simulink model "Example"  (R2025a)
settings: Solver=VariableStepAuto  StartTime=0.0  StopTime=100  RelTol=1e-3
PostLoadFcn:
  | TP_prop = Generate_TP_Prop('E:\refprop10\REFPROP','R134a',0.001,5.5,80,510,100,25,25);
  | TL_prop = Generate_TL_Prop('E:\refprop10\REFPROP','Water',0.01,50,273.16,373.16,20,20);
undefined symbols (not defined in the file): nu_liq, nu_vap, p, s_liq, s_vap, u_sat_liq, u_sat_vap
libraries: fl_lib x62, nesl_utility x34, SimscapeFluids_lib x28
(part 3 of 3)

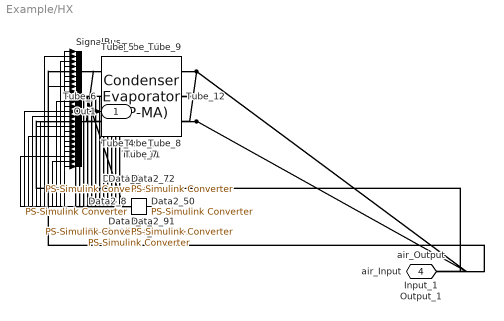
== system Example/HX ==
  Data1_{1..12} (12 alike) : nesl_utility/PS-Simulink Converter  PhysicalDomain=network_engine_domain  SubClassName=ps_output  LeftPortType=input  RightPortType=output  PseudoPeriodic=off  Frequencies=[]  VectorFormat=inherit  Unit=inherit  AffineConversion=off
  Data2_{1..12} (12 alike) : nesl_utility/PS-Simulink Converter  PhysicalDomain=network_engine_domain  SubClassName=ps_output  LeftPortType=input  RightPortType=output  PseudoPeriodic=off  Frequencies=[]  VectorFormat=inherit  Unit=inherit  AffineConversion=off
  SignalBus : BusCreator  Inputs=24
  Tube_1 : SimscapeFluids_lib/Heat Exchangers/Two-Phase Fluid - Moist Air/Condenser Evaporator (2P-MA)  flow_arrangement=fluids.heat_exchangers.enum.FlowArrangement2PMA.Cross  cross_flow_arrangement=fluids.heat_exchangers.enum.CrossFlowArrangement2PMA.UnmixedUnmixed  R_wall=1000*log(Tube_outer_diameter/Tube_inner_diameter)/(2*pi*Length_tube_segment*380) K/kW  wall_thermal_mass=false  mass_wall=1 kg  cp_wall=490 J/(K*kg)  area_A1=Cross_sectional_area_A1 m^2  area_B1=pi*Tube_inner_diameter^2/4 m^2  area_A2=Cross_sectional_area_A2/4 m^2  area_B2=Cross_sectional_area_B2/4 m^2  tube_num_2P=1  tube_length_2P=Total_length_each_tube m  tube_cross_section_2P=fluids.heat_exchangers.enum.TubeCrossSection.Circular  tube_diameter_2P=Tube_inner_diameter m  tube_width_2P=0.05 m  tube_height_2P=0.05 m  tube_inner_diameter_2P=0.05 m  tube_outer_diameter_2P=0.1 m  tube_flow_area_2P=0.002 m^2  tube_wetted_perimeter_2P=0.15 m  tube_heat_perimeter_2P=0.15 m  tube_pressure_loss_spec_2P=fluids.heat_exchangers.enum.TubePressureLossSpec2P.Haaland  tube_loss_coeff_2P=10  tube_local_pressure_loss_spec_2P=fluids.heat_exchangers.enum.LocalLossSpec.AggregateLength  tube_length_add_2P=Agg_equiv_length m  tube_local_loss_coefficient_2P=0.1  tube_roughness_pressure_2P=Internal_surface_roughness m  tube_Re_lam_pressure_2P=2000  tube_Re_tur_pressure_2P=4000  tube_shape_factor_generic_2P=64  tube_heat_coeff_spec_2P=fluids.heat_exchangers.enum.TubeHeatCoeffSpec2P.GneilinskiCavalliniZecchin  tube_colburn_coeff_liq_2P=[.023, .8, .33]  tube_colburn_coeff_mix_2P=[.05, .8, .33]  tube_colburn_coeff_vap_2P=[.023, .8, .33]  tube_roughness_heat_2P=15e-6 m  tube_Re_lam_heat_2P=2000  tube_Re_tur_heat_2P=4000  tube_Nu_lam_generic_2P=3.66  fouling_factor_2P=0.1 K*m^2/kW  fin_area_2P=0 m^2  fin_efficiency_2P=0.5  energy_spec_2P=foundation.enum.energy_spec.temperature  p_init_2P=Initial_pressure MPa  T_init_2P=Initial_temperature K  x_init_2P=0.5  alpha_init_2P=0.5  h_init_2P=1500 kJ/kg  u_init_2P=1500 kJ/kg  flow_geometry_MA=fluids.heat_exchangers.enum.FlowGeometryMA.AcrossTubeBank  tube_num_MA=25  tube_length_MA=1 m  tube_cross_section_MA=fluids.heat_exchangers.enum.TubeCrossSection.Circular  tube_diameter_MA=0.05 m  tube_width_MA=0.05 m  tube_height_MA=0.05 m  tube_inner_diameter_MA=0.05 m  tube_outer_diameter_MA=0.1 m  tube_flow_area_MA=0.002 m^2  tube_wetted_perimeter_MA=0.15 m  tube_heat_perimeter_MA=0.15 m  tube_pressure_loss_spec_MA=fluids.heat_exchangers.enum.TubePressureLossSpec.Haaland  tube_loss_coeff_MA=10  tube_local_pressure_loss_spec_MA=fluids.heat_exchangers.enum.LocalLossSpec.AggregateLength  tube_length_add_MA=0.1 m  tube_local_loss_coefficient_MA=0.1  tube_roughness_pressure_MA=15e-6 m  tube_Re_lam_pressure_MA=2000  tube_Re_tur_pressure_MA=4000  tube_shape_factor_generic_MA=64  tube_heat_coeff_spec_MA=fluids.heat_exchangers.enum.TubeHeatCoeffSpec.Gneilinski  tube_colburn_coeff_MA=[.023, .8, .33]  tube_roughness_heat_MA=15e-6 m  tube_Re_lam_heat_MA=2000  tube_Re_tur_heat_MA=4000  tube_Nu_lam_generic_MA=3.66  bank_arrangement_MA=fluids.heat_exchangers.enum.BankArrangement.Inline  bank_num_rows_MA=1  bank_tubes_per_row_MA=1  bank_width_MA=Length_tube_segment m  bank_tube_diameter_MA=Tube_outer_diameter m  bank_longitudinal_pitch_MA=Longitudinal_tube_pitch m  bank_transverse_pitch_MA=Transverse_tube_pitch m  bank_pressure_loss_spec_MA=fluids.heat_exchangers.enum.BankPressureLossSpec.Martin  bank_euler_MA=10  bank_heat_coeff_spec_MA=fluids.heat_exchangers.enum.BankHeatCoeffSpec.Martin  bank_colburn_coeff_MA=[.27, .63, .36]  generic_flow_area_MA=0.01 m^2  generic_heat_area_MA=2 m^2  generic_volume_MA=0.05 m^3  generic_loss_coeff_MA=10  generic_colburn_coeff_MA=[.023, .8, .33]  fouling_factor_MA=Fouling_factor_air K*m^2/kW  fin_area_MA=Total_fin_surface_area_air m^2  fin_efficiency_MA=Fin_efficiency_air  p_init_MA=Initial_pressure_air MPa  T_init_MA=Initial_temperature_air K  humidity_spec_MA=foundation.enum.HumiditySpec.RelativeHumidity  RH_init_MA=Initial_rel_humidity  x_w_init_MA=0.01  y_w_init_MA=0.01  HR_init_MA=0.01  Tw_init_MA=287 K  trace_gas_spec_MA=foundation.enum.trace_gas_spec.mass_fraction  x_g_init_MA=0.001  y_g_init_MA=0.001  r_d_init_MA=0  RH_ws_MA=1  time_constant_cond_MA=1e-3 s  time_constant_evap_MA=1e-3 s  fraction_entrained_MA=1
      settings: InternalSimscapePortConfiguration="{\"Bottom\":[],\"Left\":[{\"id\":\"A1\",\"label\":\"A1\",\"type\":\"foundation.two_phase_fluid.two_phase_fluid\"},{\"id\":\"Z\",\"label\":\"Z\",\"type\":\"output\"},{\"id\":\"B1\",\"label\":\"B1\",\"type\":\"foundation.two_phase_fluid.two_phase_fluid\"}],\"Right\":[{\"id\":\"A2\",\"label\":\"A2\",\"type\":\"foundation.moist_air.moist_air\"},{\"id\":\"W\",\"label\":\"W\",\"type\":\"output\"},{\"id\":\"B2\",\"label\":\"B2\",\"type\":\"foundation.moist_air.moist_air\"}],\"Top\":[]}"
  Tube_{2..11} (10 alike) : SimscapeFluids_lib/Heat Exchangers/Two-Phase Fluid - Moist Air/Condenser Evaporator (2P-MA)  flow_arrangement=fluids.heat_exchangers.enum.FlowArrangement2PMA.Cross  cross_flow_arrangement=fluids.heat_exchangers.enum.CrossFlowArrangement2PMA.UnmixedUnmixed  R_wall=1000*log(Tube_outer_diameter/Tube_inner_diameter)/(2*pi*Length_tube_segment*380) K/kW  wall_thermal_mass=false  mass_wall=1 kg  cp_wall=490 J/(K*kg)  area_A1=pi*Tube_inner_diameter^2/4 m^2  area_B1=pi*Tube_inner_diameter^2/4 m^2  area_A2=Cross_sectional_area_A2/4 m^2  area_B2=Cross_sectional_area_B2/4 m^2  tube_num_2P=1  tube_length_2P=Total_length_each_tube m  tube_cross_section_2P=fluids.heat_exchangers.enum.TubeCrossSection.Circular  tube_diameter_2P=Tube_inner_diameter m  tube_width_2P=0.05 m  tube_height_2P=0.05 m  tube_inner_diameter_2P=0.05 m  tube_outer_diameter_2P=0.1 m  tube_flow_area_2P=0.002 m^2  tube_wetted_perimeter_2P=0.15 m  tube_heat_perimeter_2P=0.15 m  tube_pressure_loss_spec_2P=fluids.heat_exchangers.enum.TubePressureLossSpec2P.Haaland  tube_loss_coeff_2P=10  tube_local_pressure_loss_spec_2P=fluids.heat_exchangers.enum.LocalLossSpec.AggregateLength  tube_length_add_2P=Agg_equiv_length m  tube_local_loss_coefficient_2P=0.1  tube_roughness_pressure_2P=Internal_surface_roughness m  tube_Re_lam_pressure_2P=2000  tube_Re_tur_pressure_2P=4000  tube_shape_factor_generic_2P=64  tube_heat_coeff_spec_2P=fluids.heat_exchangers.enum.TubeHeatCoeffSpec2P.GneilinskiCavalliniZecchin  tube_colburn_coeff_liq_2P=[.023, .8, .33]  tube_colburn_coeff_mix_2P=[.05, .8, .33]  tube_colburn_coeff_vap_2P=[.023, .8, .33]  tube_roughness_heat_2P=15e-6 m  tube_Re_lam_heat_2P=2000  tube_Re_tur_heat_2P=4000  tube_Nu_lam_generic_2P=3.66  fouling_factor_2P=0.1 K*m^2/kW  fin_area_2P=0 m^2  fin_efficiency_2P=0.5  energy_spec_2P=foundation.enum.energy_spec.temperature  p_init_2P=Initial_pressure MPa  T_init_2P=Initial_temperature K  x_init_2P=0.5  alpha_init_2P=0.5  h_init_2P=1500 kJ/kg  u_init_2P=1500 kJ/kg  flow_geometry_MA=fluids.heat_exchangers.enum.FlowGeometryMA.AcrossTubeBank  tube_num_MA=25  tube_length_MA=1 m  tube_cross_section_MA=fluids.heat_exchangers.enum.TubeCrossSection.Circular  tube_diameter_MA=0.05 m  tube_width_MA=0.05 m  tube_height_MA=0.05 m  tube_inner_diameter_MA=0.05 m  tube_outer_diameter_MA=0.1 m  tube_flow_area_MA=0.002 m^2  tube_wetted_perimeter_MA=0.15 m  tube_heat_perimeter_MA=0.15 m  tube_pressure_loss_spec_MA=fluids.heat_exchangers.enum.TubePressureLossSpec.Haaland  tube_loss_coeff_MA=10  tube_local_pressure_loss_spec_MA=fluids.heat_exchangers.enum.LocalLossSpec.AggregateLength  tube_length_add_MA=0.1 m  tube_local_loss_coefficient_MA=0.1  tube_roughness_pressure_MA=15e-6 m  tube_Re_lam_pressure_MA=2000  tube_Re_tur_pressure_MA=4000  tube_shape_factor_generic_MA=64  tube_heat_coeff_spec_MA=fluids.heat_exchangers.enum.TubeHeatCoeffSpec.Gneilinski  tube_colburn_coeff_MA=[.023, .8, .33]  tube_roughness_heat_MA=15e-6 m  tube_Re_lam_heat_MA=2000  tube_Re_tur_heat_MA=4000  tube_Nu_lam_generic_MA=3.66  bank_arrangement_MA=fluids.heat_exchangers.enum.BankArrangement.Inline  bank_num_rows_MA=1  bank_tubes_per_row_MA=1  bank_width_MA=Length_tube_segment m  bank_tube_diameter_MA=Tube_outer_diameter m  bank_longitudinal_pitch_MA=Longitudinal_tube_pitch m  bank_transverse_pitch_MA=Transverse_tube_pitch m  bank_pressure_loss_spec_MA=fluids.heat_exchangers.enum.BankPressureLossSpec.Martin  bank_euler_MA=10  bank_heat_coeff_spec_MA=fluids.heat_exchangers.enum.BankHeatCoeffSpec.Martin  bank_colburn_coeff_MA=[.27, .63, .36]  generic_flow_area_MA=0.01 m^2  generic_heat_area_MA=2 m^2  generic_volume_MA=0.05 m^3  generic_loss_coeff_MA=10  generic_colburn_coeff_MA=[.023, .8, .33]  fouling_factor_MA=Fouling_factor_air K*m^2/kW  fin_area_MA=Total_fin_surface_area_air m^2  fin_efficiency_MA=Fin_efficiency_air  p_init_MA=Initial_pressure_air MPa  T_init_MA=Initial_temperature_air K  humidity_spec_MA=foundation.enum.HumiditySpec.RelativeHumidity  RH_init_MA=Initial_rel_humidity  x_w_init_MA=0.01  y_w_init_MA=0.01  HR_init_MA=0.01  Tw_init_MA=287 K  trace_gas_spec_MA=foundation.enum.trace_gas_spec.mass_fraction  x_g_init_MA=0.001  y_g_init_MA=0.001  r_d_init_MA=0  RH_ws_MA=1  time_constant_cond_MA=1e-3 s  time_constant_evap_MA=1e-3 s  fraction_entrained_MA=1
      settings: InternalSimscapePortConfiguration="{\"Bottom\":[],\"Left\":[{\"id\":\"A1\",\"label\":\"A1\",\"type\":\"foundation.two_phase_fluid.two_phase_fluid\"},{\"id\":\"Z\",\"label\":\"Z\",\"type\":\"output\"},{\"id\":\"B1\",\"label\":\"B1\",\"type\":\"foundation.two_phase_fluid.two_phase_fluid\"}],\"Right\":[{\"id\":\"A2\",\"label\":\"A2\",\"type\":\"foundation.moist_air.moist_air\"},{\"id\":\"W\",\"label\":\"W\",\"type\":\"output\"},{\"id\":\"B2\",\"label\":\"B2\",\"type\":\"foundation.moist_air.moist_air\"}],\"Top\":[]}"
  Tube_12 : SimscapeFluids_lib/Heat Exchangers/Two-Phase Fluid - Moist Air/Condenser Evaporator (2P-MA)  flow_arrangement=fluids.heat_exchangers.enum.FlowArrangement2PMA.Cross  cross_flow_arrangement=fluids.heat_exchangers.enum.CrossFlowArrangement2PMA.UnmixedUnmixed  R_wall=1000*log(Tube_outer_diameter/Tube_inner_diameter)/(2*pi*Length_tube_segment*380) K/kW  wall_thermal_mass=false  mass_wall=1 kg  cp_wall=490 J/(K*kg)  area_A1=pi*Tube_inner_diameter^2/4 m^2  area_B1=Cross_sectional_area_B1 m^2  area_A2=Cross_sectional_area_A2/4 m^2  area_B2=Cross_sectional_area_B2/4 m^2  tube_num_2P=1  tube_length_2P=Total_length_each_tube m  tube_cross_section_2P=fluids.heat_exchangers.enum.TubeCrossSection.Circular  tube_diameter_2P=Tube_inner_diameter m  tube_width_2P=0.05 m  tube_height_2P=0.05 m  tube_inner_diameter_2P=0.05 m  tube_outer_diameter_2P=0.1 m  tube_flow_area_2P=0.002 m^2  tube_wetted_perimeter_2P=0.15 m  tube_heat_perimeter_2P=0.15 m  tube_pressure_loss_spec_2P=fluids.heat_exchangers.enum.TubePressureLossSpec2P.Haaland  tube_loss_coeff_2P=10  tube_local_pressure_loss_spec_2P=fluids.heat_exchangers.enum.LocalLossSpec.AggregateLength  tube_length_add_2P=Agg_equiv_length m  tube_local_loss_coefficient_2P=0.1  tube_roughness_pressure_2P=Internal_surface_roughness m  tube_Re_lam_pressure_2P=2000  tube_Re_tur_pressure_2P=4000  tube_shape_factor_generic_2P=64  tube_heat_coeff_spec_2P=fluids.heat_exchangers.enum.TubeHeatCoeffSpec2P.GneilinskiCavalliniZecchin  tube_colburn_coeff_liq_2P=[.023, .8, .33]  tube_colburn_coeff_mix_2P=[.05, .8, .33]  tube_colburn_coeff_vap_2P=[.023, .8, .33]  tube_roughness_heat_2P=15e-6 m  tube_Re_lam_heat_2P=2000  tube_Re_tur_heat_2P=4000  tube_Nu_lam_generic_2P=3.66  fouling_factor_2P=0.1 K*m^2/kW  fin_area_2P=0 m^2  fin_efficiency_2P=0.5  energy_spec_2P=foundation.enum.energy_spec.temperature  p_init_2P=Initial_pressure MPa  T_init_2P=Initial_temperature K  x_init_2P=0.5  alpha_init_2P=0.5  h_init_2P=1500 kJ/kg  u_init_2P=1500 kJ/kg  flow_geometry_MA=fluids.heat_exchangers.enum.FlowGeometryMA.AcrossTubeBank  tube_num_MA=25  tube_length_MA=1 m  tube_cross_section_MA=fluids.heat_exchangers.enum.TubeCrossSection.Circular  tube_diameter_MA=0.05 m  tube_width_MA=0.05 m  tube_height_MA=0.05 m  tube_inner_diameter_MA=0.05 m  tube_outer_diameter_MA=0.1 m  tube_flow_area_MA=0.002 m^2  tube_wetted_perimeter_MA=0.15 m  tube_heat_perimeter_MA=0.15 m  tube_pressure_loss_spec_MA=fluids.heat_exchangers.enum.TubePressureLossSpec.Haaland  tube_loss_coeff_MA=10  tube_local_pressure_loss_spec_MA=fluids.heat_exchangers.enum.LocalLossSpec.AggregateLength  tube_length_add_MA=0.1 m  tube_local_loss_coefficient_MA=0.1  tube_roughness_pressure_MA=15e-6 m  tube_Re_lam_pressure_MA=2000  tube_Re_tur_pressure_MA=4000  tube_shape_factor_generic_MA=64  tube_heat_coeff_spec_MA=fluids.heat_exchangers.enum.TubeHeatCoeffSpec.Gneilinski  tube_colburn_coeff_MA=[.023, .8, .33]  tube_roughness_heat_MA=15e-6 m  tube_Re_lam_heat_MA=2000  tube_Re_tur_heat_MA=4000  tube_Nu_lam_generic_MA=3.66  bank_arrangement_MA=fluids.heat_exchangers.enum.BankArrangement.Inline  bank_num_rows_MA=1  bank_tubes_per_row_MA=1  bank_width_MA=Length_tube_segment m  bank_tube_diameter_MA=Tube_outer_diameter m  bank_longitudinal_pitch_MA=Longitudinal_tube_pitch m  bank_transverse_pitch_MA=Transverse_tube_pitch m  bank_pressure_loss_spec_MA=fluids.heat_exchangers.enum.BankPressureLossSpec.Martin  bank_euler_MA=10  bank_heat_coeff_spec_MA=fluids.heat_exchangers.enum.BankHeatCoeffSpec.Martin  bank_colburn_coeff_MA=[.27, .63, .36]  generic_flow_area_MA=0.01 m^2  generic_heat_area_MA=2 m^2  generic_volume_MA=0.05 m^3  generic_loss_coeff_MA=10  generic_colburn_coeff_MA=[.023, .8, .33]  fouling_factor_MA=Fouling_factor_air K*m^2/kW  fin_area_MA=Total_fin_surface_area_air m^2  fin_efficiency_MA=Fin_efficiency_air  p_init_MA=Initial_pressure_air MPa  T_init_MA=Initial_temperature_air K  humidity_spec_MA=foundation.enum.HumiditySpec.RelativeHumidity  RH_init_MA=Initial_rel_humidity  x_w_init_MA=0.01  y_w_init_MA=0.01  HR_init_MA=0.01  Tw_init_MA=287 K  trace_gas_spec_MA=foundation.enum.trace_gas_spec.mass_fraction  x_g_init_MA=0.001  y_g_init_MA=0.001  r_d_init_MA=0  RH_ws_MA=1  time_constant_cond_MA=1e-3 s  time_constant_evap_MA=1e-3 s  fraction_entrained_MA=1
      settings: InternalSimscapePortConfiguration="{\"Bottom\":[],\"Left\":[{\"id\":\"A1\",\"label\":\"A1\",\"type\":\"foundation.two_phase_fluid.two_phase_fluid\"},{\"id\":\"Z\",\"label\":\"Z\",\"type\":\"output\"},{\"id\":\"B1\",\"label\":\"B1\",\"type\":\"foundation.two_phase_fluid.two_phase_fluid\"}],\"Right\":[{\"id\":\"A2\",\"label\":\"A2\",\"type\":\"foundation.moist_air.moist_air\"},{\"id\":\"W\",\"label\":\"W\",\"type\":\"output\"},{\"id\":\"B2\",\"label\":\"B2\",\"type\":\"foundation.moist_air.moist_air\"}],\"Top\":[]}"
  Input_1 : PMIOPort  Side=Left
  Output_1 : PMIOPort  Port=2  Side=Left
  air_Input : PMIOPort  Port=3  Side=Left
  air_Output : PMIOPort  Port=4  Side=Left
  Out1 : Outport
  wires:
  Data1_1/1 -> SignalBus/1
  Data1_2/1 -> SignalBus/3
  Data1_6/1 -> SignalBus/11
  Data1_12/1 -> SignalBus/23
  Data2_4/1 -> SignalBus/8
  SignalBus/1 -> Out1/1
  Data2_1/1 -> SignalBus/2
  Data1_8/1 -> SignalBus/15
  Data2_8/1 -> SignalBus/16
  Data2_7/1 -> SignalBus/14
  Data2_9/1 -> SignalBus/18
  Data1_7/1 -> SignalBus/13
  Data2_11/1 -> SignalBus/22
  Data1_11/1 -> SignalBus/21
  Data2_6/1 -> SignalBus/12
  Data2_12/1 -> SignalBus/24
  Data1_4/1 -> SignalBus/7
  Data2_3/1 -> SignalBus/6
  Data2_5/1 -> SignalBus/10
  Data1_5/1 -> SignalBus/9
  Data1_3/1 -> SignalBus/5
  Data2_2/1 -> SignalBus/4
  Data1_9/1 -> SignalBus/17
  Data2_10/1 -> SignalBus/20
  Data1_10/1 -> SignalBus/19
  connections:
  Tube_3/LConn3 -- Tube_6/LConn1
  Tube_6/RConn1 -- Tube_5/RConn3
  Tube_5/RConn1 -- Tube_4/RConn3
  Tube_11/RConn1 -- Tube_10/RConn3
  Input_1/RConn1 -- Tube_1/LConn1
  Tube_8/RConn2 -- Data2_8/LConn1
  Tube_7/LConn2 -- Data1_7/LConn1
  Tube_7/LConn3 -- Tube_10/LConn1
  Tube_8/LConn2 -- Data1_8/LConn1
  Tube_6/RConn2 -- Data2_6/LConn1
  Tube_1/RConn1 -- air_Input/RConn1 -- Tube_10/RConn1 -- Tube_7/RConn1 -- Tube_4/RConn1
  Output_1/RConn1 -- Tube_12/LConn3
  Tube_7/RConn2 -- Data2_7/LConn1
  Tube_5/LConn3 -- Tube_2/LConn1
  Tube_12/RConn2 -- Data2_12/LConn1
  Tube_9/RConn1 -- Tube_8/RConn3
  Tube_5/LConn2 -- Data1_5/LConn1
  Tube_3/RConn1 -- Tube_2/RConn3
  Tube_12/LConn2 -- Data1_12/LConn1
  Tube_6/LConn2 -- Data1_6/LConn1
  Tube_6/LConn3 -- Tube_9/LConn1
  Tube_3/RConn3 -- air_Output/RConn1 -- Tube_12/RConn3 -- Tube_9/RConn3 -- Tube_6/RConn3
  Tube_11/RConn2 -- Data2_11/LConn1
  Tube_1/LConn3 -- Tube_4/LConn1
  Tube_9/RConn2 -- Data2_9/LConn1
  Tube_10/LConn3 -- Tube_11/LConn1
  Tube_11/LConn2 -- Data1_11/LConn1
  Tube_8/RConn1 -- Tube_7/RConn3
  Tube_4/LConn2 -- Data1_4/LConn1
  Tube_4/LConn3 -- Tube_7/LConn1
  Tube_4/RConn2 -- Data2_4/LConn1
  Tube_2/RConn1 -- Tube_1/RConn3
  Tube_12/RConn1 -- Tube_11/RConn3
  Tube_5/RConn2 -- Data2_5/LConn1
  Tube_3/RConn2 -- Data2_3/LConn1
  Tube_3/LConn2 -- Data1_3/LConn1
  Tube_9/LConn3 -- Tube_12/LConn1
  Tube_2/LConn3 -- Tube_3/LConn1
  Tube_8/LConn3 -- Tube_5/LConn1
  Tube_11/LConn3 -- Tube_8/LConn1
  Tube_9/LConn2 -- Data1_9/LConn1
  Tube_1/LConn2 -- Data1_1/LConn1
  Tube_10/RConn2 -- Data2_10/LConn1
  Tube_10/LConn2 -- Data1_10/LConn1
  Tube_1/RConn2 -- Data2_1/LConn1
  Tube_2/RConn2 -- Data2_2/LConn1
  Tube_2/LConn2 -- Data1_2/LConn1
